simulink model "PID_Controller"  (R2018b)
settings: Solver=ode23s  StartTime=0.0  StopTime=10.0  RelTol=1e-3  AbsTol=AUTO  EnableMultiTasking=on
undefined symbols (not defined in the file or in its folder): Fmatrix, Imatrix
libraries: dspinverses x1
(part 3 of 5)

== matlab function PID_Controller/MANIPULARTOR/Subsystem1/Gravity Vector/G_matrix ==
  data: in1 input; G output
function G = Gmatrix(in1)

G=zeros(6,1);
%GMATRIX
%    G = GMATRIX(IN1)

%    This function was generated by the Symbolic Math Toolbox version 7.0.
%    08-Aug-2017 18:04:37

q2 = in1(2,:);
q3 = in1(3,:);
q4 = in1(4,:);
q5 = in1(5,:);
t2 = sin(q2);
t3 = cos(q2);
t4 = cos(q3);
t5 = sin(q3);
t6 = t2.*t5;
t7 = cos(q5);
t8 = t3.*t5;
t9 = t2.*t4;
t10 = t8+t9;
t11 = sin(q4);
t15 = t3.*t4;
t12 = t6-t15;
t13 = cos(q4);
t14 = sin(q5);
G = [0.0;t2.*(-4.742496)-t7.*t10.*1.0978e-1-t11.*t12.*3.481024+t12.*t13.*t14.*1.0978e-1;t7.*t10.*(-1.0978e-1)-t11.*t12.*3.481024+t13.*t14.*(t6-t15).*1.0978e-1;t10.*t13.*3.481024+t10.*t11.*t14.*1.0978e-1;t14.*(t6-t15).*1.0978e-1-t7.*t10.*t13.*1.0978e-1;0.0];

== matlab function PID_Controller/MATLAB Function ==
  data: theta1 input; X output; theta2 input; theta3 input; theta4 input; theta5 input; theta6 input; Y output; Z output
function [X,Y,Z]=ForwardKinematic(theta1,theta2,theta3,theta4,theta5,theta6)

A01 = [ cosd(theta1)  0    -sind(theta1)    0;
        sind(theta1)  0     cosd(theta1)    0;
        0                -1     0                   0;
        0                 0     0                   1;];
 
A12 = [ cosd(theta2)  -sind(theta2)   0     0.5*cosd(theta2);
        sind(theta2)   cosd(theta2)   0     0.5*sind(theta2);
        0                  0                  1     0.25;
        0                  0                  0     1;];  
    
A23 = [ cosd(theta3)  0    sind(theta3)    0;
        sind(theta3)  0   -cosd(theta3)    0;
        0                 1     0                  0;
        0                 0     0                  1;];    

A34 = [ cosd(theta4)  0   -sind(theta4)    0;
        sind(theta4)  0    cosd(theta4)    0;
        0                -1     0                  1;
        0                 0     0                  1;];  

A45 = [ cosd(theta5)  0    sind(theta5)    0;
        sind(theta5)  0   -cosd(theta5)    0;
        0                 1     0                  0;
        0                 0     0                  1;];    
    
A56 = [ cosd(theta6)  -sind(theta6)   0     0;
        sind(theta6)   cosd(theta6)   0     0;
        0                  0                  1     0.5;
        0                  0                  0     1;];  
 
F1 = A01*A12*A23*A34*A45*A56;

%% Result
X = F1(1,4);
Y = F1(2,4);
Z = F1(3,4);
